simulink model "uav_control"  (R2023b)
settings: Solver=ode45  StartTime=0  StopTime=1000  RelTol=1e-4
values from neighbouring files (symbols this model uses):
  b = 2.9    [config.m]
  c = 0.19    [config.m]
  C_D = [0.043, 0.030, 0, 0.0135]    [config.m]
  C_l = [0 , -0.13, -0.51, 0.25, 0.17, 0.0024]    [config.m]
  C_L = [0.23, 5.61, 7.95, 0.13]    [config.m]
  C_m = [0.0135, -2.74, -38.21, -0.99]    [config.m]
  C_n = [0, 0.073, -0.069, -0.095, -0.011, -0.069]    [config.m]
  C_Q = [C_q2, C_q1, C_q0]    [config.m]
  C_T = [C_t2, C_t1, C_t0]    [config.m]
  C_Y = [0, -0.83, 0, 0, 0.075, 0.19]    [config.m]
  D = 0.508    [config.m]
  i_0 = 1.5    [config.m]
  K_Q = 0.0659    [config.m]
  K_V = 0.0659    [config.m]
  mass = 11    [config.m]
  p = 1.268    [config.m]
  R_motor = 0.042    [config.m]
  S = 0.55    [config.m]
  V_max = 44.4    [config.m]
undefined symbols (not defined in the file or in its folder): Aileron, alpha, beta, Elevator, gamma, Rudder, Throttle, Va
undefined symbols (not defined in the file): F_b, M_b
libraries: sharedtransform x2, shared6dof x1
settings Model: PauseTimes=0  Creator=Victor  LastModifiedBy=Victor
settings DataIOCC: ExternalInput=getinputstruct(op2)  InitialState=getstatestruct(op2)
settings DebuggingCC: MaxConsecutiveZCsMsg=none

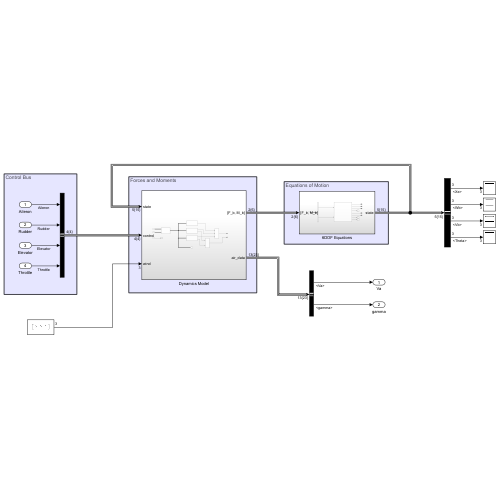
[thumbnail: Simulink's stored preview of the top-level diagram]
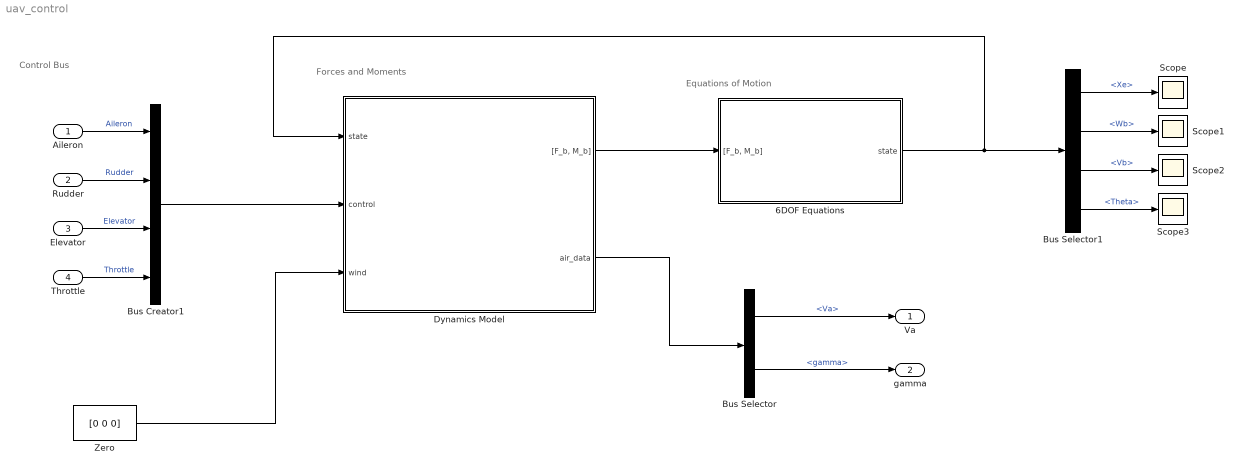
== system uav_control ==
  note: Control Bus
  note: Forces and Moments
  note: Equations of Motion
  Aileron : Inport
  Rudder : Inport  Port=2
  Elevator : Inport  Port=3
  Throttle : Inport  Port=4
  6DOF Equations : Subsystem
  Bus Creator1 : BusCreator  Inputs=Aileron,Rudder,Elevator,Throttle
  Bus Selector : BusSelector  OutputSignals=target.Va,target.gamma
  Bus Selector1 : BusSelector  OutputSignals=Xe,Wb,Vb,Theta
  Dynamics Model : Subsystem
  Scope{,1..3} (4 alike) : Scope
  Zero : Constant  Value=[0 0 0]
  Va : Outport
  gamma : Outport  Port=2
  wires:
  6DOF Equations/1(state) -> Dynamics Model/1(state), Bus Selector1/1
  Aileron/1 -> Bus Creator1/1  "Aileron"
  Rudder/1 -> Bus Creator1/2  "Rudder"
  Elevator/1 -> Bus Creator1/3  "Elevator"
  Throttle/1 -> Bus Creator1/4  "Throttle"
  Dynamics Model/1("[F_b, M_b]") -> 6DOF Equations/1("[F_b, M_b]")
  Bus Creator1/1 -> Dynamics Model/2(control)
  Dynamics Model/2(air_data) -> Bus Selector/1
  Zero/1 -> Dynamics Model/3(wind)
  Bus Selector/1 -> Va/1  "<Va>"
  Bus Selector/2 -> gamma/1  "<gamma>"
  Bus Selector1/1 -> Scope/1  "<Xe>"
  Bus Selector1/2 -> Scope1/1  "<Wb>"
  Bus Selector1/3 -> Scope2/1  "<Vb>"
  Bus Selector1/4 -> Scope3/1  "<Theta>"

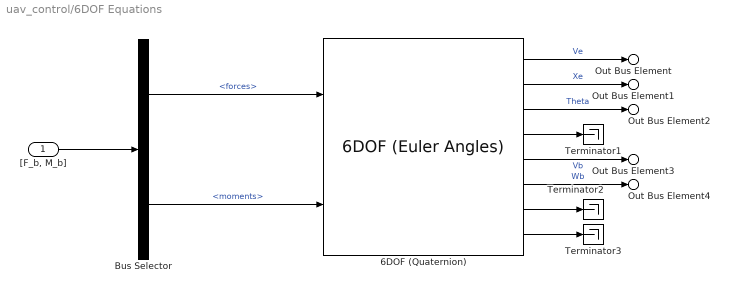
== system uav_control/6DOF Equations ==
  "[F_b, M_b]" : Inport
  6DOF (Quaternion) : shared6dof/6DOF (Euler Angles)  units=Metric (MKS)  mtype=Fixed  rep=Euler Angles  xme_0=x_0  Vm_0=v_0  eul_0=theta_0  pm_0=w_0  mass_0=mass  mass_e=0.5  mass_f=2.0  inertia=I  inertia_e=eye(3)  inertia_f=2*eye(3)  k_quat=1.0  vre_flag=on  abi_flag=off  aMode=0  xme_statename=''  Vm_statename=''  eul_statename=''  quat_statename=''  pm_statename=''  mass_statename=''
      settings: LibrarySourceBlock=aerolib6dof2/6DOF (Quaternion)
  Bus Selector : BusSelector  OutputSignals=forces,moments
  Terminator1 : Terminator
  Terminator2 : Terminator
  Terminator3 : Terminator
  Out Bus Element : Outport  PortName=state  Element=Ve
  Out Bus Element1 : Outport  PortName=state  Element=Xe
  Out Bus Element2 : Outport  PortName=state  Element=Theta
  Out Bus Element3 : Outport  PortName=state  Element=Vb
  Out Bus Element4 : Outport  PortName=state  Element=Wb
  wires:
  6DOF (Quaternion)/8 -> Terminator3/1
  6DOF (Quaternion)/4 -> Terminator1/1
  6DOF (Quaternion)/7 -> Terminator2/1
  "[F_b, M_b]"/1 -> Bus Selector/1
  Bus Selector/1 -> 6DOF (Quaternion)/1  "<forces>"
  Bus Selector/2 -> 6DOF (Quaternion)/2  "<moments>"
  6DOF (Quaternion)/1 -> Out Bus Element/1  "Ve"
  6DOF (Quaternion)/2 -> Out Bus Element1/1  "Xe"
  6DOF (Quaternion)/3 -> Out Bus Element2/1  "Theta"
  6DOF (Quaternion)/5 -> Out Bus Element3/1  "Vb"
  6DOF (Quaternion)/6 -> Out Bus Element4/1  "Wb"

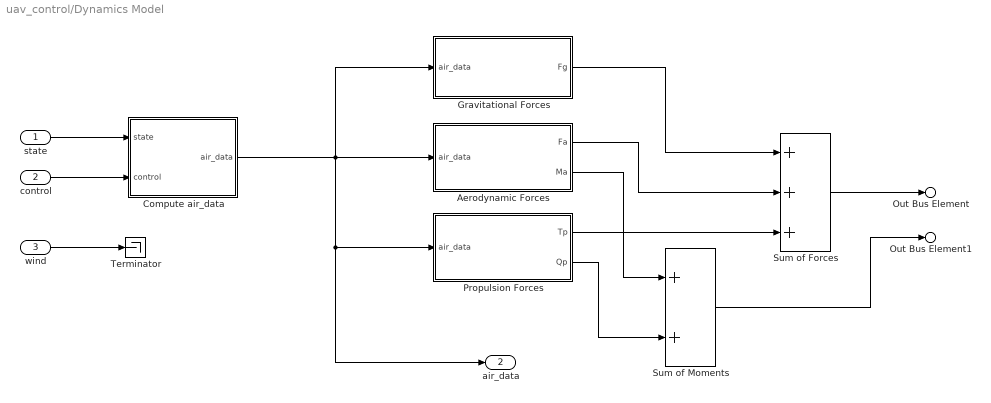
== system uav_control/Dynamics Model ==
  state : Inport
  control : Inport  Port=2
  wind : Inport  Port=3
  Aerodynamic Forces : Subsystem
  Compute air_data : Subsystem
  Gravitational Forces : Subsystem
  Propulsion Forces : Subsystem
  Sum of Forces : Sum  Inputs=+++
  Sum of Moments : Sum
  Terminator : Terminator
  Out Bus Element : Outport  PortName=[F_b, M_b]  Element=forces
  Out Bus Element1 : Outport  PortName=[F_b, M_b]  Element=moments
  air_data : Outport  Port=2
  wires:
  Aerodynamic Forces/2(Ma) -> Sum of Moments/1
  Propulsion Forces/2(Qp) -> Sum of Moments/2
  Propulsion Forces/1(Tp) -> Sum of Forces/3
  Aerodynamic Forces/1(Fa) -> Sum of Forces/2
  Gravitational Forces/1(Fg) -> Sum of Forces/1
  Sum of Moments/1 -> Out Bus Element1/1
  Sum of Forces/1 -> Out Bus Element/1
  wind/1 -> Terminator/1
  state/1 -> Compute air_data/1(state)
  control/1 -> Compute air_data/2(control)
  Compute air_data/1(air_data) -> Propulsion Forces/1(air_data), air_data/1, Gravitational Forces/1(air_data), Aerodynamic Forces/1(air_data)

== system uav_control/Dynamics Model/Aerodynamic Forces ==
  air_data : Inport
  Add : Sum
  Add1 : Sum
  Lateral Forces : Subsystem
  Longitudinal Forces : Subsystem
  Fa : Outport
  Ma : Outport  Port=2
  wires:
  Add1/1 -> Ma/1
  Longitudinal Forces/2(Ma_b) -> Add1/2
  Lateral Forces/2(MaL_b) -> Add1/1
  Add/1 -> Fa/1
  Longitudinal Forces/1(fa_b) -> Add/2
  Lateral Forces/1(faL_b) -> Add/1
  air_data/1 -> Longitudinal Forces/1(air_data), Lateral Forces/1(air_data)

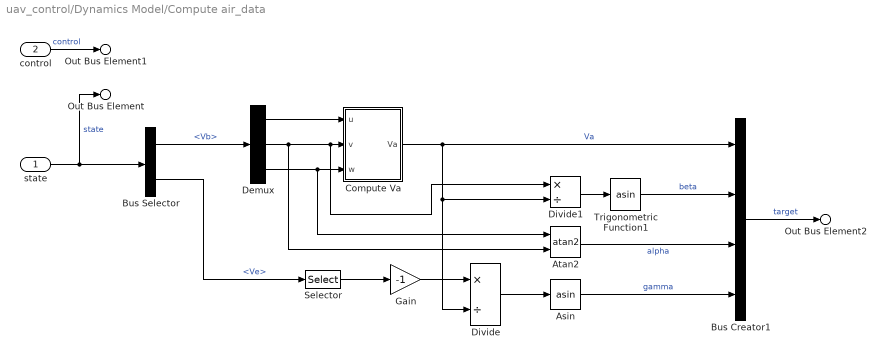
== system uav_control/Dynamics Model/Compute air_data ==
  state : Inport
  control : Inport  Port=2
  Asin : Trigonometry  Operator=asin
  Atan2 : Trigonometry  Operator=atan2
  Bus Creator1 : BusCreator  Inputs=Va,beta,alpha,gamma
  Bus Selector : BusSelector  OutputSignals=Vb,Ve
  Compute Va : Subsystem
  Demux : Demux  Outputs=3
  Divide : Product  Inputs=*/
  Divide1 : Product  Inputs=*/
  Gain : Gain  Gain=-1
  Selector : Selector  InputPortWidth=3  IndexOptions=Index vector (dialog)  Indices=[2]  OutputSizes=1
  Trigonometric Function1 : Trigonometry  Operator=asin
  Out Bus Element : Outport  PortName=air_data  Element=state
  Out Bus Element1 : Outport  PortName=air_data  Element=control
  Out Bus Element2 : Outport  PortName=air_data  Element=target
  wires:
  state/1 -> Out Bus Element/1, Bus Selector/1  "state"
  Trigonometric Function1/1 -> Bus Creator1/2  "beta"
  Divide1/1 -> Trigonometric Function1/1
  Compute Va/1(Va) -> Bus Creator1/1, Divide1/2, Divide/2  "Va"
  Atan2/1 -> Bus Creator1/3  "alpha"
  Demux/2 -> Divide1/1, Compute Va/2(v), Atan2/2
  Demux/1 -> Compute Va/1(u)
  Bus Creator1/1 -> Out Bus Element2/1  "target"
  control/1 -> Out Bus Element1/1  "control"
  Selector/1 -> Gain/1
  Gain/1 -> Divide/1
  Divide/1 -> Asin/1
  Bus Selector/1 -> Demux/1  "<Vb>"
  Asin/1 -> Bus Creator1/4  "gamma"
  Demux/3 -> Compute Va/3(w), Atan2/1
  Bus Selector/2 -> Selector/1  "<Ve>"

== system uav_control/Dynamics Model/Gravitational Forces ==
  air_data : Inport
  Bus Selector : BusSelector  OutputSignals=state.Theta
  Gravity : Gain  Gain=9.81
  Mass : Constant  Value=mass
  Vector Concatenate : Concatenate  NumInputs=3
  Vehicle-frame to Body-frame : Subsystem
  Zero : Constant  Value=0  OutDataTypeStr=Inherit: Inherit via back propagation
  Fg : Outport
  wires:
  Mass/1 -> Gravity/1
  Gravity/1 -> Vector Concatenate/3
  Zero/1 -> Vector Concatenate/1, Vector Concatenate/2
  Vector Concatenate/1 -> Vehicle-frame to Body-frame/2(Fg_v)  "Fg_v"
  Vehicle-frame to Body-frame/1(Fg_b) -> Fg/1
  air_data/1 -> Bus Selector/1
  Bus Selector/1 -> Vehicle-frame to Body-frame/1(Theta)  "<Theta>"

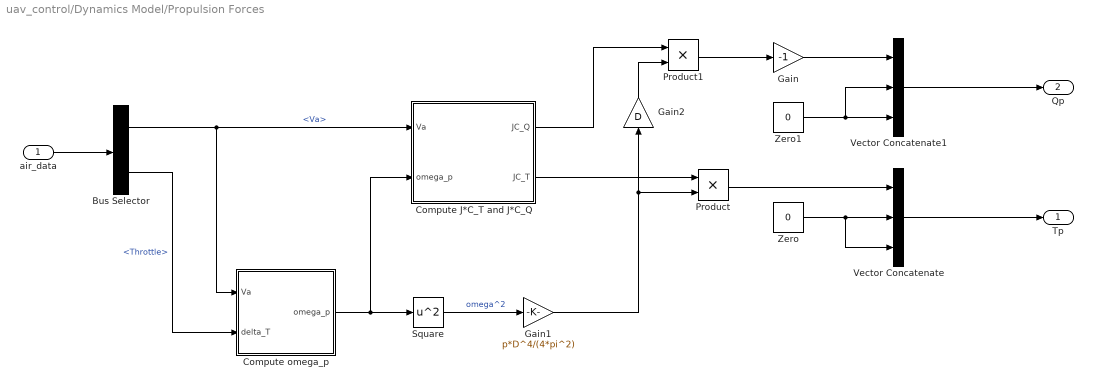
== system uav_control/Dynamics Model/Propulsion Forces ==
  air_data : Inport
  Bus Selector : BusSelector  OutputSignals=target.Va,control.Throttle
  Compute J*C_T and J*C_Q : Subsystem
  Compute omega_p : Subsystem
  Gain : Gain  Gain=-1
  Gain1 : Gain  Gain=p*D^4/(4*pi^2)
  Gain2 : Gain  Gain=D
  Product : Product
  Product1 : Product
  Square : Math  Operator=square
  Vector Concatenate : Concatenate  NumInputs=3
  Vector Concatenate1 : Concatenate  NumInputs=3
  Zero : Constant  Value=0  OutDataTypeStr=Inherit: Inherit via back propagation
  Zero1 : Constant  Value=0  OutDataTypeStr=Inherit: Inherit via back propagation
  Tp : Outport
  Qp : Outport  Port=2
  wires:
  Zero/1 -> Vector Concatenate/2, Vector Concatenate/3
  Vector Concatenate/1 -> Tp/1
  Zero1/1 -> Vector Concatenate1/2, Vector Concatenate1/3
  Vector Concatenate1/1 -> Qp/1
  Gain/1 -> Vector Concatenate1/1
  air_data/1 -> Bus Selector/1
  Product/1 -> Vector Concatenate/1
  Product1/1 -> Gain/1
  Gain1/1 -> Gain2/1, Product/2
  Square/1 -> Gain1/1  "omega^2"
  Compute omega_p/1(omega_p) -> Compute J*C_T and J*C_Q/2(omega_p), Square/1
  Bus Selector/1 -> Compute J*C_T and J*C_Q/1(Va), Compute omega_p/1(Va)  "<Va>"
  Compute J*C_T and J*C_Q/2(JC_T) -> Product/1
  Compute J*C_T and J*C_Q/1(JC_Q) -> Product1/1
  Bus Selector/2 -> Compute omega_p/2(delta_T)  "<Throttle>"
  Gain2/1 -> Product1/2

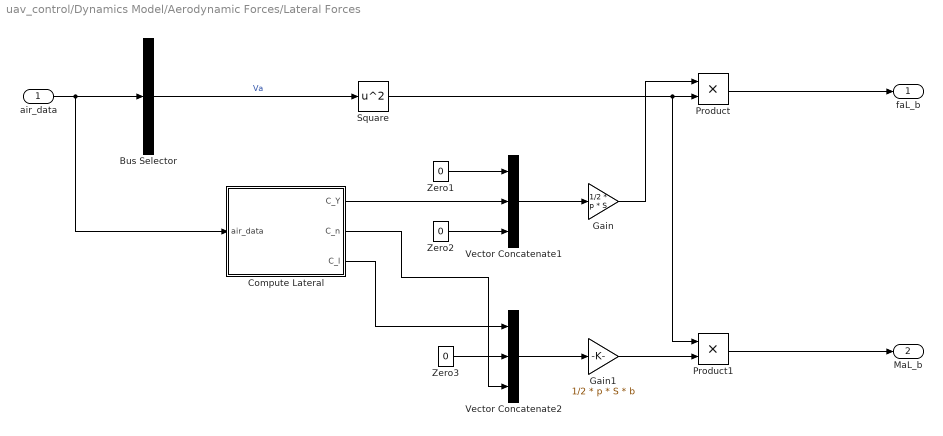
== system uav_control/Dynamics Model/Aerodynamic Forces/Lateral Forces ==
  air_data : Inport
  Bus Selector : BusSelector  OutputSignals=target.Va  OutputAsBus=on
  Compute Lateral : Subsystem
  Gain : Gain  Gain=1/2 * p * S
  Gain1 : Gain  Gain=1/2 * p * S * b
  Product : Product
  Product1 : Product
  Square : Math  Operator=square
  Vector Concatenate1 : Concatenate  NumInputs=3
  Vector Concatenate2 : Concatenate  NumInputs=3
  Zero1 : Constant  Value=0  OutDataTypeStr=Inherit: Inherit via back propagation
  Zero2 : Constant  Value=0  OutDataTypeStr=Inherit: Inherit via back propagation
  Zero3 : Constant  Value=0  OutDataTypeStr=Inherit: Inherit via back propagation
  faL_b : Outport
  MaL_b : Outport  Port=2
  wires:
  Vector Concatenate1/1 -> Gain/1
  Bus Selector/1 -> Square/1  "Va"
  Product1/1 -> MaL_b/1
  Vector Concatenate2/1 -> Gain1/1
  Product/1 -> faL_b/1
  air_data/1 -> Compute Lateral/1(air_data), Bus Selector/1
  Gain1/1 -> Product1/2
  Gain/1 -> Product/1
  Zero1/1 -> Vector Concatenate1/1
  Zero2/1 -> Vector Concatenate1/3
  Compute Lateral/1(C_Y) -> Vector Concatenate1/2
  Compute Lateral/2(C_n) -> Vector Concatenate2/3
  Compute Lateral/3(C_l) -> Vector Concatenate2/1
  Square/1 -> Product1/1, Product/2
  Zero3/1 -> Vector Concatenate2/2

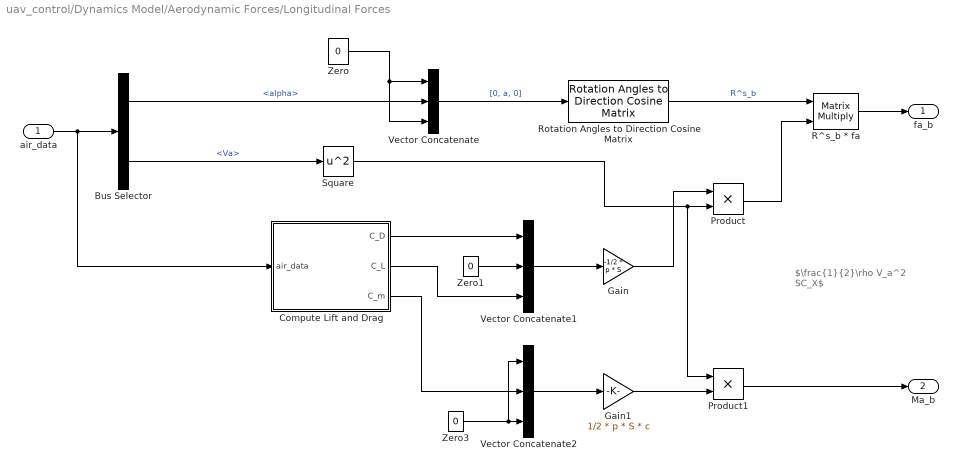
== system uav_control/Dynamics Model/Aerodynamic Forces/Longitudinal Forces ==
  note: $\frac{1}{2}\rho V_a^2 SC_X$
  air_data : Inport
  Bus Selector : BusSelector  OutputSignals=target.alpha,target.Va
  Compute Lift and Drag : Subsystem
  Gain : Gain  Gain=-1/2 * p * S
  Gain1 : Gain  Gain=1/2 * p * S * c
  Product : Product
  Product1 : Product
  R^s_b * fa : Product  Multiplication=Matrix(*)
  Rotation Angles to Direction Cosine Matrix : sharedtransform/Rotation Angles to Direction Cosine Matrix  rotationOrder=ZYX  aMode=aMode
  Square : Math  Operator=square
  Vector Concatenate : Concatenate  NumInputs=3
  Vector Concatenate1 : Concatenate  NumInputs=3
  Vector Concatenate2 : Concatenate  NumInputs=3
  Zero : Constant  Value=0  OutDataTypeStr=Inherit: Inherit via back propagation
  Zero1 : Constant  Value=0  OutDataTypeStr=Inherit: Inherit via back propagation
  Zero3 : Constant  Value=0  OutDataTypeStr=Inherit: Inherit via back propagation
  fa_b : Outport
  Ma_b : Outport  Port=2
  wires:
  Vector Concatenate/1 -> Rotation Angles to Direction Cosine Matrix/1  "[0, a, 0]"
  Zero/1 -> Vector Concatenate/3, Vector Concatenate/1
  Rotation Angles to Direction Cosine Matrix/1 -> R^s_b * fa/1  "R^s_b"
  air_data/1 -> Bus Selector/1, Compute Lift and Drag/1(air_data)
  Vector Concatenate1/1 -> Gain/1
  Zero1/1 -> Vector Concatenate1/2
  R^s_b * fa/1 -> fa_b/1
  Gain/1 -> Product/1
  Compute Lift and Drag/1(C_D) -> Vector Concatenate1/1
  Compute Lift and Drag/2(C_L) -> Vector Concatenate1/3
  Product/1 -> R^s_b * fa/2
  Vector Concatenate2/1 -> Gain1/1
  Zero3/1 -> Vector Concatenate2/1, Vector Concatenate2/3
  Compute Lift and Drag/3(C_m) -> Vector Concatenate2/2
  Gain1/1 -> Product1/2
  Product1/1 -> Ma_b/1
  Square/1 -> Product/2, Product1/1
  Bus Selector/1 -> Vector Concatenate/2  "<alpha>"
  Bus Selector/2 -> Square/1  "<Va>"

== system uav_control/Dynamics Model/Compute air_data/Compute Va ==
  u : Inport
  v : Inport  Port=2
  w : Inport  Port=3
  Add : Sum  Inputs=+++
  Square : Math  Operator=square
  Square Root : Sqrt
  Square1 : Math  Operator=square
  Square2 : Math  Operator=square
  Va : Outport
  wires:
  Square2/1 -> Add/3
  Square/1 -> Add/1
  Add/1 -> Square Root/1
  Square1/1 -> Add/2
  u/1 -> Square/1
  w/1 -> Square2/1
  v/1 -> Square1/1
  Square Root/1 -> Va/1  "Va"

== system uav_control/Dynamics Model/Gravitational Forces/Vehicle-frame to Body-frame ==
  Theta : Inport
  Fg_v : Inport  Port=2
  Display : Display
  Display1 : Display
  Matrix Multiply : Product  Multiplication=Matrix(*)
  R^v_b : sharedtransform/Rotation Angles to Direction Cosine Matrix  rotationOrder=ZYX  aMode=aMode
  Selector : Selector  InputPortWidth=3  IndexOptions=Index vector (dialog)  Indices=[3 2 1]  OutputSizes=1
  Fg_b : Outport
  wires:
  Matrix Multiply/1 -> Fg_b/1
  Theta/1 -> Display/1, Selector/1
  Selector/1 -> Display1/1, R^v_b/1
  R^v_b/1 -> Matrix Multiply/1
  Fg_v/1 -> Matrix Multiply/2

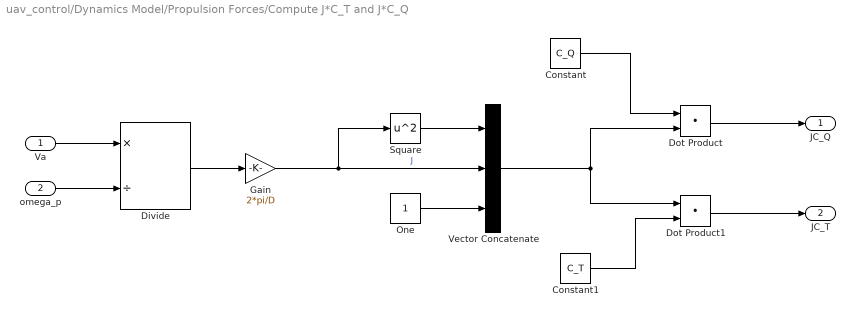
== system uav_control/Dynamics Model/Propulsion Forces/Compute J*C_T and J*C_Q ==
  Va : Inport
  omega_p : Inport  Port=2
  Constant : Constant  Value=C_Q
  Constant1 : Constant  Value=C_T
  Divide : Product  Inputs=*/
  Dot Product : DotProduct  OutDataTypeStr=Inherit: Inherit via internal rule
  Dot Product1 : DotProduct  OutDataTypeStr=Inherit: Inherit via internal rule
  Gain : Gain  Gain=2*pi/D
  One : Constant  OutDataTypeStr=Inherit: Inherit via back propagation
  Square : Math  Operator=square
  Vector Concatenate : Concatenate  NumInputs=3
  JC_Q : Outport
  JC_T : Outport  Port=2
  wires:
  Va/1 -> Divide/1
  omega_p/1 -> Divide/2
  Divide/1 -> Gain/1
  Gain/1 -> Square/1, Vector Concatenate/2  "J"
  Square/1 -> Vector Concatenate/1
  One/1 -> Vector Concatenate/3
  Constant/1 -> Dot Product/1
  Vector Concatenate/1 -> Dot Product1/1, Dot Product/2
  Constant1/1 -> Dot Product1/2
  Dot Product1/1 -> JC_T/1
  Dot Product/1 -> JC_Q/1

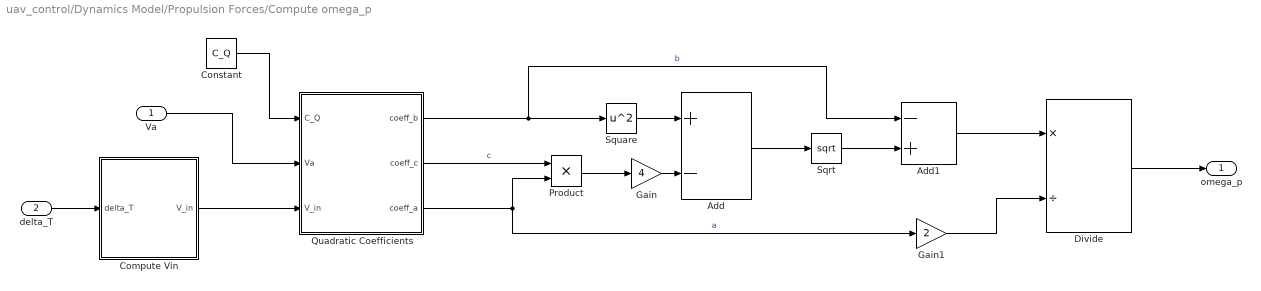
== system uav_control/Dynamics Model/Propulsion Forces/Compute omega_p ==
  Va : Inport
  delta_T : Inport  Port=2
  Add : Sum  Inputs=+-
  Add1 : Sum  Inputs=-+
  Compute Vin : Subsystem
  Constant : Constant  Value=C_Q
  Divide : Product  Inputs=*/
  Gain : Gain  Gain=4
  Gain1 : Gain  Gain=2
  Product : Product
  Quadratic Coefficients : Subsystem
  Sqrt : Sqrt
  Square : Math  Operator=square
  omega_p : Outport
  wires:
  delta_T/1 -> Compute Vin/1(delta_T)
  Constant/1 -> Quadratic Coefficients/1(C_Q)
  Square/1 -> Add/1
  Gain/1 -> Add/2
  Product/1 -> Gain/1
  Add/1 -> Sqrt/1
  Gain1/1 -> Divide/2
  Divide/1 -> omega_p/1
  Quadratic Coefficients/1(coeff_b) -> Add1/1, Square/1  "b"
  Quadratic Coefficients/2(coeff_c) -> Product/1  "c"
  Quadratic Coefficients/3(coeff_a) -> Gain1/1, Product/2  "a"
  Sqrt/1 -> Add1/2
  Add1/1 -> Divide/1
  Va/1 -> Quadratic Coefficients/2(Va)
  Compute Vin/1(V_in) -> Quadratic Coefficients/3(V_in)

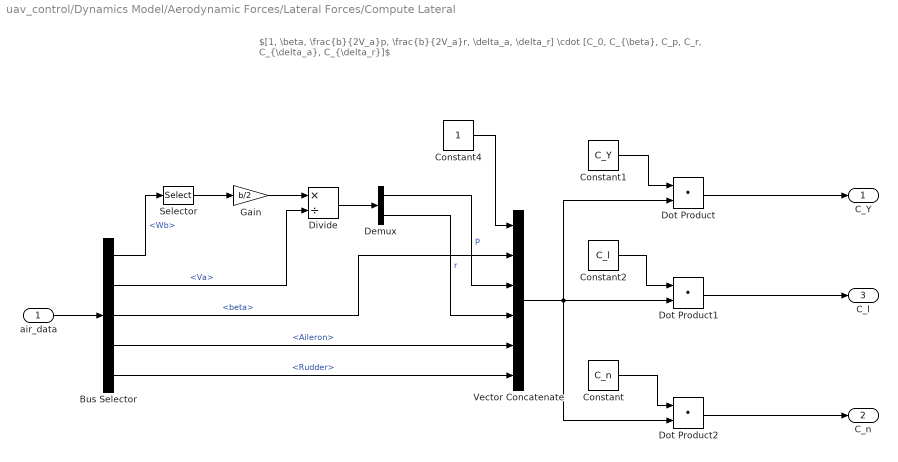
== system uav_control/Dynamics Model/Aerodynamic Forces/Lateral Forces/Compute Lateral ==
  note: $[1, \beta, \frac{b}{2V_a}p, \frac{b}{2V_a}r, \delta_a, \delta_r] \cdot [C_0, C_{\beta}, C_p, C_r, C_{\delta_a}, C_{\delta_r}]$
  air_data : Inport
  Bus Selector : BusSelector  OutputSignals=state.Wb,target.Va,target.beta,control.Aileron,control.Rudder
  Constant : Constant  Value=C_n
  Constant1 : Constant  Value=C_Y
  Constant2 : Constant  Value=C_l
  Constant4 : Constant
  Demux : Demux  Outputs=2
  Divide : Product  Inputs=*/
  Dot Product : DotProduct  OutDataTypeStr=Inherit: Inherit via internal rule
  Dot Product1 : DotProduct  OutDataTypeStr=Inherit: Inherit via internal rule
  Dot Product2 : DotProduct  OutDataTypeStr=Inherit: Inherit via internal rule
  Gain : Gain  Gain=b/2
  Selector : Selector  InputPortWidth=3  IndexOptions=Index vector (dialog)  Indices=[1 3]  OutputSizes=1
  Vector Concatenate : Concatenate  NumInputs=6
  C_Y : Outport
  C_n : Outport  Port=2
  C_l : Outport  Port=3
  wires:
  air_data/1 -> Bus Selector/1
  Constant1/1 -> Dot Product/1
  Vector Concatenate/1 -> Dot Product2/2, Dot Product1/2, Dot Product/2
  Constant2/1 -> Dot Product1/1
  Dot Product/1 -> C_Y/1
  Dot Product1/1 -> C_l/1
  Dot Product2/1 -> C_n/1
  Gain/1 -> Divide/1
  Constant4/1 -> Vector Concatenate/1
  Demux/1 -> Vector Concatenate/3  "p"
  Demux/2 -> Vector Concatenate/4  "r"
  Divide/1 -> Demux/1
  Constant/1 -> Dot Product2/1
  Selector/1 -> Gain/1
  Bus Selector/1 -> Selector/1  "<Wb>"
  Bus Selector/2 -> Divide/2  "<Va>"
  Bus Selector/3 -> Vector Concatenate/2  "<beta>"
  Bus Selector/4 -> Vector Concatenate/5  "<Aileron>"
  Bus Selector/5 -> Vector Concatenate/6  "<Rudder>"

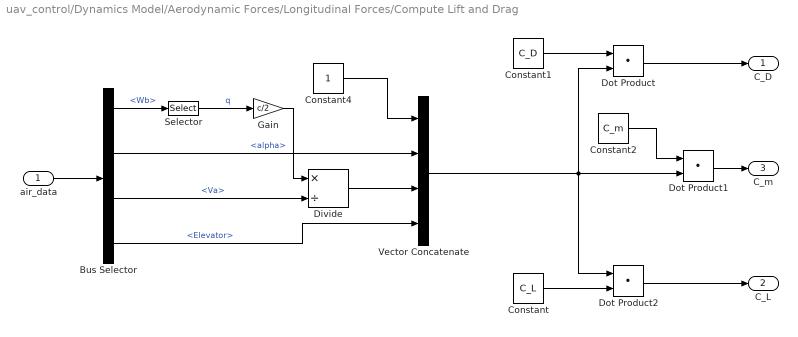
== system uav_control/Dynamics Model/Aerodynamic Forces/Longitudinal Forces/Compute Lift and Drag ==
  air_data : Inport
  Bus Selector : BusSelector  OutputSignals=state.Wb,target.alpha,target.Va,control.Elevator
  Constant : Constant  Value=C_L
  Constant1 : Constant  Value=C_D
  Constant2 : Constant  Value=C_m
  Constant4 : Constant
  Divide : Product  Inputs=*/
  Dot Product : DotProduct  OutDataTypeStr=Inherit: Inherit via internal rule
  Dot Product1 : DotProduct  OutDataTypeStr=Inherit: Inherit via internal rule
  Dot Product2 : DotProduct  OutDataTypeStr=Inherit: Inherit via internal rule
  Gain : Gain  Gain=c/2
  Selector : Selector  InputPortWidth=3  IndexOptions=Index vector (dialog)  Indices=[2]  OutputSizes=1
  Vector Concatenate : Concatenate  NumInputs=4
  C_D : Outport
  C_L : Outport  Port=2
  C_m : Outport  Port=3
  wires:
  Constant4/1 -> Vector Concatenate/1
  air_data/1 -> Bus Selector/1
  Bus Selector/2 -> Vector Concatenate/2  "<alpha>"
  Bus Selector/3 -> Divide/2  "<Va>"
  Gain/1 -> Divide/1
  Divide/1 -> Vector Concatenate/3
  Bus Selector/4 -> Vector Concatenate/4  "<Elevator>"
  Constant1/1 -> Dot Product/1
  Vector Concatenate/1 -> Dot Product2/1, Dot Product1/2, Dot Product/2
  Constant/1 -> Dot Product2/2
  Constant2/1 -> Dot Product1/1
  Dot Product/1 -> C_D/1
  Dot Product1/1 -> C_m/1
  Dot Product2/1 -> C_L/1
  Selector/1 -> Gain/1  "q"
  Bus Selector/1 -> Selector/1  "<Wb>"

== system uav_control/Dynamics Model/Propulsion Forces/Compute omega_p/Compute Vin ==
  delta_T : Inport
  Constant : Constant  Value=0.5
  Manual Switch : ManualSwitch
  Product : Product
  V_max : Constant  Value=V_max
  V_in : Outport
  wires:
  delta_T/1 -> Manual Switch/1
  V_max/1 -> Product/2
  Product/1 -> V_in/1
  Manual Switch/1 -> Product/1
  Constant/1 -> Manual Switch/2

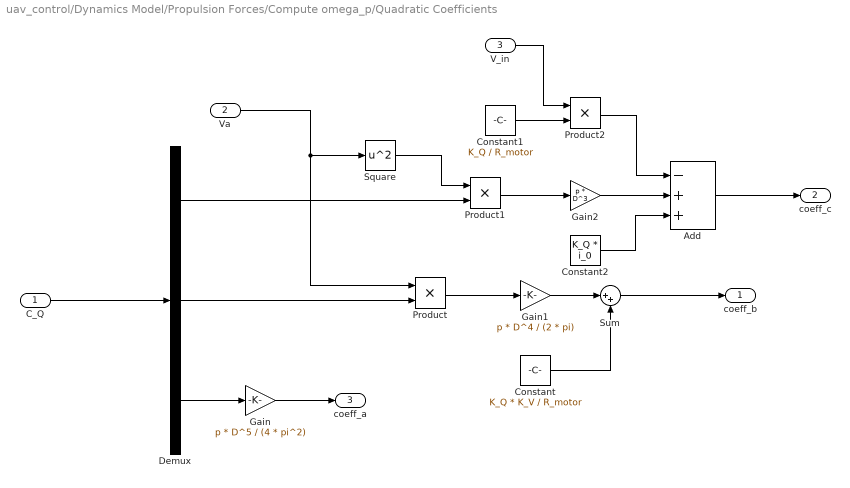
== system uav_control/Dynamics Model/Propulsion Forces/Compute omega_p/Quadratic Coefficients ==
  C_Q : Inport
  Va : Inport  Port=2
  V_in : Inport  Port=3
  Add : Sum  Inputs=-++
  Constant : Constant  Value=K_Q * K_V / R_motor
  Constant1 : Constant  Value=K_Q / R_motor
  Constant2 : Constant  Value=K_Q * i_0
  Demux : Demux  Outputs=3
  Gain : Gain  Gain=p * D^5 / (4 * pi^2)
  Gain1 : Gain  Gain=p * D^4 / (2 * pi)
  Gain2 : Gain  Gain=p * D^3
  Product : Product
  Product1 : Product
  Product2 : Product
  Square : Math  Operator=square
  Sum : Sum  Inputs=|++
  coeff_b : Outport
  coeff_c : Outport  Port=2
  coeff_a : Outport  Port=3
  wires:
  Gain/1 -> coeff_a/1
  C_Q/1 -> Demux/1
  Demux/3 -> Gain/1
  Demux/2 -> Product/2
  Va/1 -> Square/1, Product/1
  Product/1 -> Gain1/1
  Gain1/1 -> Sum/1
  Constant/1 -> Sum/2
  Sum/1 -> coeff_b/1
  Product1/1 -> Gain2/1
  Square/1 -> Product1/1
  Demux/1 -> Product1/2
  Gain2/1 -> Add/2
  Constant2/1 -> Add/3
  Constant1/1 -> Product2/2
  V_in/1 -> Product2/1
  Product2/1 -> Add/1
  Add/1 -> coeff_c/1
